simulink model "model2"  (R2024b)
settings: Solver=VariableStepAuto  StartTime=0.0  StopTime=10.0  RelTol=1e-3
libraries: simulink x2
settings Model: Creator=Mehmet  LastModifiedBy=Mehmet

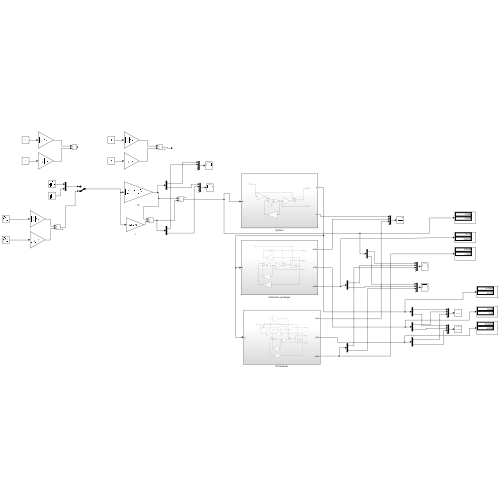
[thumbnail: Simulink's stored preview of the top-level diagram]
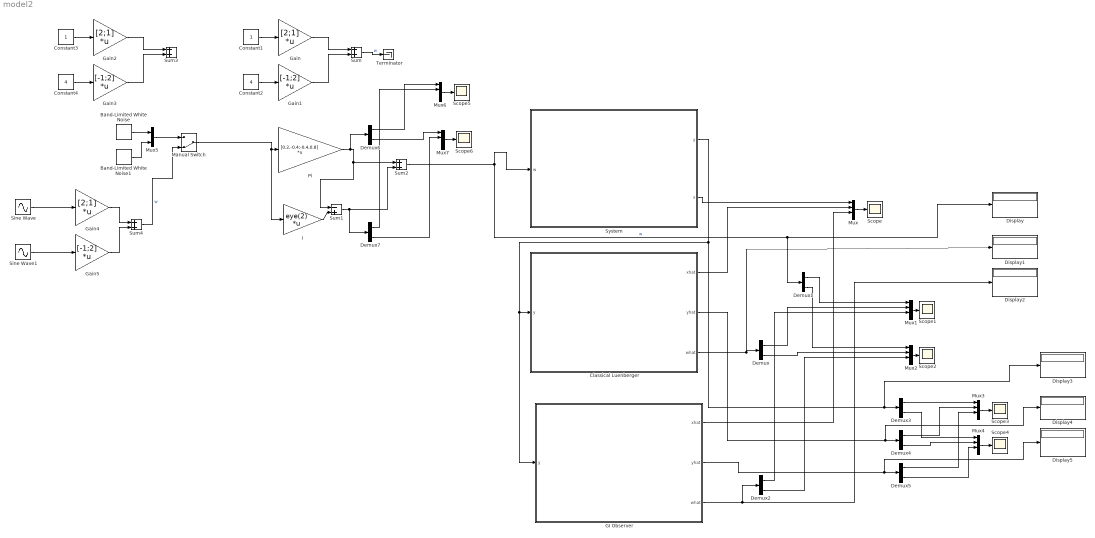
== system model2 ==
  Band-Limited White Noise : simulink/Sources/Band-Limited White Noise  Cov=[0.1]  Ts=0.1  seed=[23341]
  Band-Limited White Noise1 : simulink/Sources/Band-Limited White Noise  Cov=[0.1]  Ts=0.1  seed=[23333]
  Classical Luenberger : Subsystem
  Constant1 : Constant  VectorParams1D=off
  Constant2 : Constant  Value=4  VectorParams1D=off
  Constant3 : Constant  VectorParams1D=off
  Constant4 : Constant  Value=4  VectorParams1D=off
  Demux{,1..7} (8 alike) : Demux  Outputs=2
  Display{,1..5} (6 alike) : Display
  GI Observer : Subsystem
  Gain : Gain  Gain=[2;1]  Multiplication=Matrix(K*u)
  Gain1 : Gain  Gain=[-1;2]  Multiplication=Matrix(K*u)
  Gain2 : Gain  Gain=[2;1]  Multiplication=Matrix(K*u)
  Gain3 : Gain  Gain=[-1;2]  Multiplication=Matrix(K*u)
  Gain4 : Gain  Gain=[2;1]  Multiplication=Matrix(K*u)
  Gain5 : Gain  Gain=[-1;2]  Multiplication=Matrix(K*u)
  I : Gain  Gain=eye(2)  Multiplication=Matrix(K*u)
  Manual Switch : ManualSwitch  CurrentSetting=0
  Mux{,1..4,6..7} (7 alike) : Mux
  Mux5 : Mux  Inputs=2
  Pi : Gain  Gain=[0.2,-0.4;-0.4,0.8]  Multiplication=Matrix(K*u)
  Scope{,1..6} (7 alike) : Scope
  Sine Wave : Sin  SampleTime=0
  Sine Wave1 : Sin  Phase=pi/2  SampleTime=0
  Sum{,2..4} (4 alike) : Sum
  Sum1 : Sum  Inputs=-+
  System : Subsystem
  Terminator : Terminator
  wires:
  Constant1/1 -> Gain/1
  Constant2/1 -> Gain1/1
  Gain/1 -> Sum/1
  Gain1/1 -> Sum/2
  Sum2/1 -> System/1(w), Demux1/1, Display/1  "w"
  System/1(y) -> Display3/1, Demux3/1, GI Observer/1(y), Classical Luenberger/1(y)
  Mux/1 -> Scope/1
  System/2(x) -> Mux/1
  Mux1/1 -> Scope1/1
  Classical Luenberger/3(what) -> Demux/1, Display1/1
  GI Observer/1(xhat) -> Mux/3
  GI Observer/3(what) -> Demux2/1, Display2/1
  Mux2/1 -> Scope2/1
  Demux1/1 -> Mux1/1
  Demux1/2 -> Mux2/1
  Demux/1 -> Mux1/2
  Demux/2 -> Mux2/2
  Demux2/1 -> Mux1/3
  Demux2/2 -> Mux2/3
  Mux3/1 -> Scope3/1
  Mux4/1 -> Scope4/1
  Classical Luenberger/2(yhat) -> Display4/1, Demux4/1
  GI Observer/2(yhat) -> Display5/1, Demux5/1
  Demux3/1 -> Mux3/1
  Demux4/1 -> Mux3/2
  Demux5/1 -> Mux3/3
  Demux3/2 -> Mux4/1
  Demux4/2 -> Mux4/2
  Demux5/2 -> Mux4/3
  Classical Luenberger/1(xhat) -> Mux/2
  Manual Switch/1 -> I/1, Pi/1
  Pi/1 -> Demux6/1, Sum2/1, Sum1/1
  Sum1/1 -> Demux7/1, Sum2/2
  I/1 -> Sum1/2
  Sum/1 -> Terminator/1  "w"
  Band-Limited White Noise/1 -> Mux5/1
  Band-Limited White Noise1/1 -> Mux5/2
  Mux6/1 -> Scope5/1
  Demux6/1 -> Mux6/1
  Demux7/1 -> Mux6/2
  Mux7/1 -> Scope6/1
  Demux6/2 -> Mux7/1
  Demux7/2 -> Mux7/2
  Mux5/1 -> Manual Switch/1
  Constant3/1 -> Gain2/1
  Constant4/1 -> Gain3/1
  Gain2/1 -> Sum3/1
  Gain3/1 -> Sum3/2
  Gain4/1 -> Sum4/1
  Gain5/1 -> Sum4/2
  Sum4/1 -> Manual Switch/2  "w"
  Sine Wave/1 -> Gain4/1
  Sine Wave1/1 -> Gain5/1

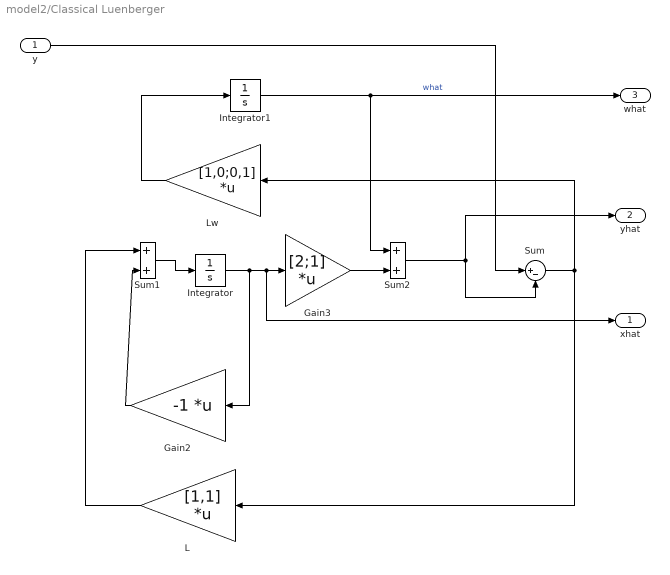
== system model2/Classical Luenberger ==
  y : Inport
  Gain2 : Gain  Gain=-1  Multiplication=Matrix(K*u)
  Gain3 : Gain  Gain=[2;1]  Multiplication=Matrix(K*u)
  Integrator : Integrator
  Integrator1 : Integrator
  L : Gain  Gain=[1,1]  Multiplication=Matrix(K*u)
  Lw : Gain  Gain=[1,0;0,1]  Multiplication=Matrix(K*u)
  Sum : Sum  Inputs=|+-
  Sum1 : Sum
  Sum2 : Sum
  xhat : Outport
  yhat : Outport  Port=2
  what : Outport  Port=3
  wires:
  Integrator/1 -> Gain2/1, xhat/1, Gain3/1
  Sum1/1 -> Integrator/1
  Sum2/1 -> yhat/1, Sum/2
  L/1 -> Sum1/1
  y/1 -> Sum/1
  Sum/1 -> Lw/1, L/1
  Gain2/1 -> Sum1/2
  Lw/1 -> Integrator1/1
  Gain3/1 -> Sum2/2
  Integrator1/1 -> Sum2/1, what/1  "what"

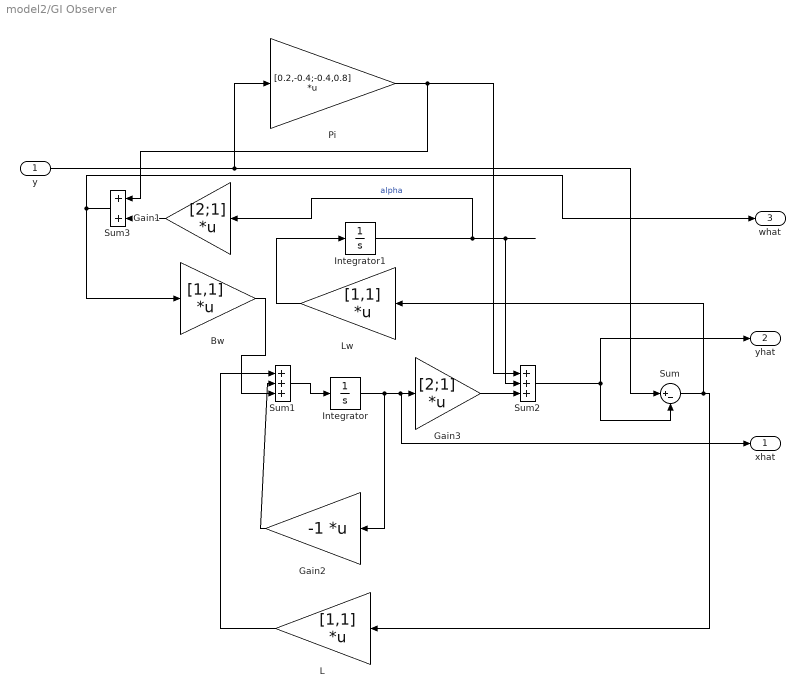
== system model2/GI Observer ==
  y : Inport
  Bw : Gain  Gain=[1,1]  Multiplication=Matrix(K*u)
  Gain1 : Gain  Gain=[2;1]  Multiplication=Matrix(K*u)
  Gain2 : Gain  Gain=-1  Multiplication=Matrix(K*u)
  Gain3 : Gain  Gain=[2;1]  Multiplication=Matrix(K*u)
  Integrator : Integrator
  Integrator1 : Integrator
  L : Gain  Gain=[1,1]  Multiplication=Matrix(K*u)
  Lw : Gain  Gain=[1,1]  Multiplication=Matrix(K*u)
  Pi : Gain  Gain=[0.2,-0.4;-0.4,0.8]  Multiplication=Matrix(K*u)
  Sum : Sum  Inputs=|+-
  Sum1 : Sum  Inputs=+++
  Sum2 : Sum  Inputs=+++
  Sum3 : Sum
  xhat : Outport
  yhat : Outport  Port=2
  what : Outport  Port=3
  wires:
  Integrator/1 -> Gain2/1, xhat/1, Gain3/1
  Sum1/1 -> Integrator/1
  Sum2/1 -> yhat/1, Sum/2
  L/1 -> Sum1/1
  y/1 -> Pi/1, Sum/1
  Sum/1 -> Lw/1, L/1
  Gain2/1 -> Sum1/2
  Lw/1 -> Integrator1/1
  Gain3/1 -> Sum2/3
  Integrator1/1 -> Gain1/1, Sum2/2  "alpha"
  Pi/1 -> Sum3/1, Sum2/1
  Bw/1 -> Sum1/3
  Gain1/1 -> Sum3/2
  Sum3/1 -> Bw/1, what/1

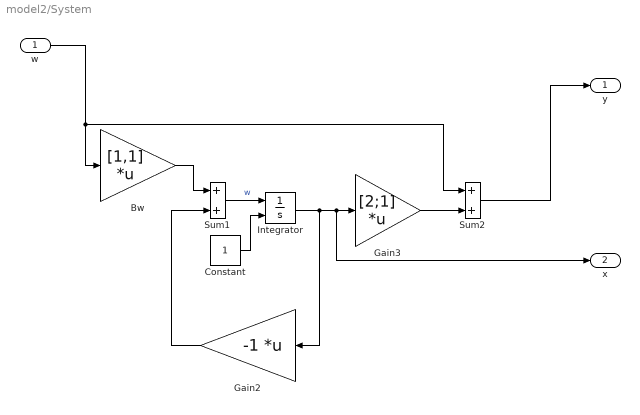
== system model2/System ==
  w : Inport
  Bw : Gain  Gain=[1,1]  Multiplication=Matrix(K*u)
  Constant : Constant  VectorParams1D=off
  Gain2 : Gain  Gain=-1  Multiplication=Matrix(K*u)
  Gain3 : Gain  Gain=[2;1]  Multiplication=Matrix(K*u)
  Integrator : Integrator  InitialConditionSource=external
  Sum1 : Sum
  Sum2 : Sum
  y : Outport
  x : Outport  Port=2
  wires:
  Sum2/1 -> y/1
  Constant/1 -> Integrator/2
  Gain3/1 -> Sum2/2
  Integrator/1 -> Gain2/1, x/1, Gain3/1
  Gain2/1 -> Sum1/2
  Bw/1 -> Sum1/1
  Sum1/1 -> Integrator/1  "w"
  w/1 -> Sum2/1, Bw/1
